simulink model "sfcndemo_hg_gui"  (Simulink 7.6)
settings: Solver=FixedStepDiscrete  StartTime=0.0  StopTime=inf  RelTol=1e-3
Description:
  | Attaching a MATLAB GUI to a Block as its Parameter Dialog for a C-MEX S-function
settings Model: Creator=The MathWorks Inc.  ExtModeTrigMode=oneshot  ExtModeArmWhenConnect=off  ExtModeAutoUpdateStatusClock=off
settings DataIOCC: LimitDataPoints=off
settings OptimizationCC: BlockReduction=off  BooleanDataType=off  InitFltsAndDblsToZero=on
settings DebuggingCC: SaveWithParameterizedLinksMsg=none  SignalResolutionControl=TryResolveAllWithWarning  SolverPrmCheckMsg=none  MultiTaskDSMMsg=warning  MultiTaskCondExecSysMsg=none
settings HardwareCC: TargetUnknown=on
settings RTWCC: IncludeERTFirstTime=on
settings CodeAppCC: CustomSymbolStrFcn=$F$N$M
settings GRTTargetCC: TargetFcnLib=ansi_tfl_tmw.mat

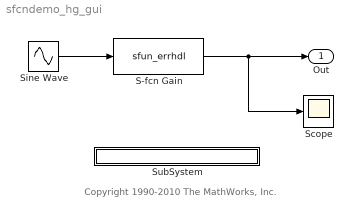
== system sfcndemo_hg_gui ==
  note: Copyright 1990-2010 The MathWorks, Inc.
  S-fcn Gain : S-Function  FunctionName=sfun_errhdl  Parameters=param  EnableBusSupport=off  mask(S-function: sfun_errhdl){param=2.3}
      mask prompts: param "Input parameter:"
      mask help: An example of handling parameter checking in S-function.
      settings: DeleteFcn=sfcndemo_hg_gui_m('delete',gcbh)  NameChangeFcn=sfcndemo_hg_gui_m('namechange',gcbh)  DestroyFcn=sfcndemo_hg_gui_m('destroy',gcbh)  OpenFcn=sfcndemo_hg_gui_m('open',gcbh)  CloseFcn=sfcndemo_hg_gui_m('close',gcbh)  ParentCloseFcn=sfcndemo_hg_gui_m('parentclose',gcbh)
      mask Display: disp('HG GUI Demo');
  Scope : Scope
      settings: TickLabels=on  TimeRange=10  YMin=-10  YMax=10  DataFormat=Array
  Sine Wave : Sin  SampleTime=0
  SubSystem : Subsystem
      settings: OpenFcn=edit('sfcndemo_hg_gui_m.m')
      mask Display: disp('Edit sfcndemo_hg_gui.m');
  Out : Outport  InitialOutput=0
  wires:
  Sine Wave/1 -> S-fcn Gain/1
  S-fcn Gain/1 -> Out/1, Scope/1

== system sfcndemo_hg_gui/SubSystem ==
